simulink model "agrivoltaics_v1"  (R2025b)
settings: Solver=FixedStepAuto  StartTime=0.0  StopTime=0  FixedStep=1  RelTol=1e-3
values from neighbouring files (symbols this model uses):
  agriParams =     [agrivoltaic_multiobjective_GA_main_data.mat]    (also in agrivoltaic_multiobjective_GA_main_data_2p7_deep.mat; agrivoltaic_multiobjective_GA_main_data_berry_pop100.mat; agrivoltaic_multiobjective_GA_main_data_berry_pop50.mat; agrivoltaic_multiobjective_GA_main_data_berry_pop80.mat)
  agriVar =     [agrivoltaic_multiobjective_GA_main_data.mat]    (also in agrivoltaic_multiobjective_GA_main_data_2p7_deep.mat; agrivoltaic_multiobjective_GA_main_data_berry_pop100.mat; agrivoltaic_multiobjective_GA_main_data_berry_pop50.mat; agrivoltaic_multiobjective_GA_main_data_berry_pop80.mat)
libraries: crop_cost x1, crop_performance_module x1, environmental_module x1, pv_performance_module x1, value x1
settings Model: Creator=ciepm  LastModifiedBy=aodha

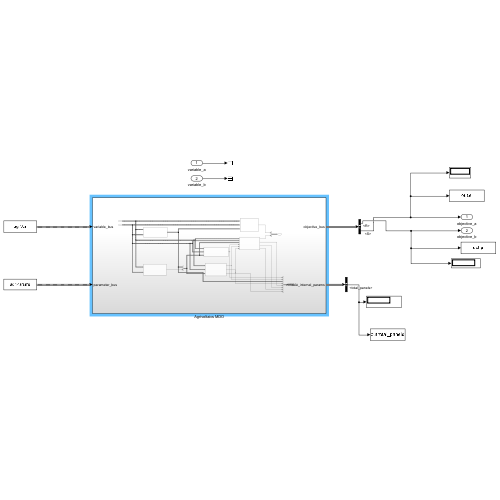
[thumbnail: Simulink's stored preview of the top-level diagram]
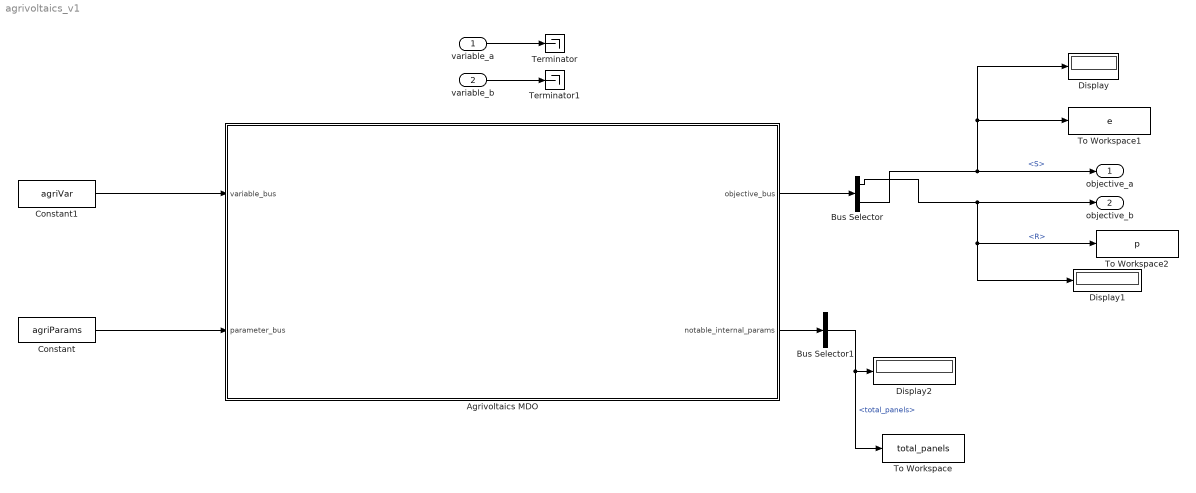
== system agrivoltaics_v1 ==
  variable_a : Inport
  variable_b : Inport  Port=2
  Agrivoltaics MDO : Subsystem
  Bus Selector : BusSelector  OutputSignals=R,S
  Bus Selector1 : BusSelector  OutputSignals=energy_per_year.total_panels
  Constant : Constant  Value=agriParams  OutDataTypeStr=Bus: params_bus
  Constant1 : Constant  Value=agriVar  OutDataTypeStr=Bus: var_bus
  Display : Display
  Display1 : Display
  Display2 : Display
  Terminator : Terminator
  Terminator1 : Terminator
  To Workspace : ToWorkspace  VariableName=total_panels  SaveFormat=Timeseries  SampleTime=-1
  To Workspace1 : ToWorkspace  VariableName=e  SaveFormat=Timeseries  SampleTime=-1
  To Workspace2 : ToWorkspace  VariableName=p  SaveFormat=Timeseries  SampleTime=-1
  objective_a : Outport
  objective_b : Outport  Port=2
  wires:
  Agrivoltaics MDO/1(objective_bus) -> Bus Selector/1
  Bus Selector/2 -> objective_a/1, To Workspace1/1, Display/1  "<S>"
  Bus Selector/1 -> objective_b/1, To Workspace2/1, Display1/1  "<R>"
  variable_a/1 -> Terminator/1
  variable_b/1 -> Terminator1/1
  Constant1/1 -> Agrivoltaics MDO/1(variable_bus)
  Agrivoltaics MDO/2(notable_internal_params) -> Bus Selector1/1
  Bus Selector1/1 -> Display2/1, To Workspace/1  "<total_panels>"
  Constant/1 -> Agrivoltaics MDO/2(parameter_bus)

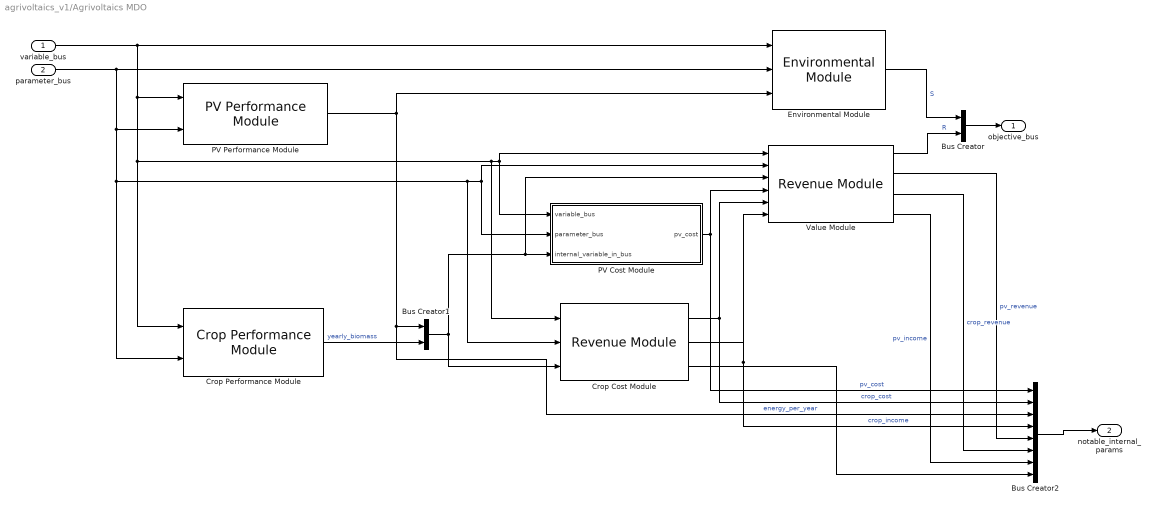
== system agrivoltaics_v1/Agrivoltaics MDO ==
  variable_bus : Inport
  parameter_bus : Inport  Port=2
  Bus Creator : BusCreator  Inputs=2
  Bus Creator1 : BusCreator  Inputs=2
  Bus Creator2 : BusCreator  Inputs=8
  Crop Cost Module : crop_cost/Revenue Module  SystemSampleTime=-1  VariantActivationTime=update diagram  EmptyChoice=off  PassThrough=off  PassThroughVariantControl=(default)  EmptyChoiceVariantControl=(default)  AllowFlexibleInterface=on  Latency=0  AutoFrameSizeCalculation=off
  Crop Performance Module : crop_performance_module/Crop Performance Module  SystemSampleTime=-1  VariantActivationTime=update diagram  EmptyChoice=off  PassThrough=off  PassThroughVariantControl=(default)  EmptyChoiceVariantControl=(default)  AllowFlexibleInterface=on  Latency=0  AutoFrameSizeCalculation=off
  Environmental Module : environmental_module/Environmental Module  SystemSampleTime=-1  VariantActivationTime=update diagram  EmptyChoice=off  PassThrough=off  PassThroughVariantControl=(default)  EmptyChoiceVariantControl=(default)  AllowFlexibleInterface=on  Latency=0  AutoFrameSizeCalculation=off
  PV Cost Module : Subsystem  AncestorBlock=pv_cost/Revenue Module
  PV Performance Module : pv_performance_module/PV Performance Module  SystemSampleTime=-1  VariantActivationTime=update diagram  EmptyChoice=off  PassThrough=off  PassThroughVariantControl=(default)  EmptyChoiceVariantControl=(default)  AllowFlexibleInterface=on  Latency=0  AutoFrameSizeCalculation=off
  Value Module : value/Revenue Module  SystemSampleTime=-1  VariantActivationTime=update diagram  EmptyChoice=off  PassThrough=off  PassThroughVariantControl=(default)  EmptyChoiceVariantControl=(default)  AllowFlexibleInterface=on  Latency=0  AutoFrameSizeCalculation=off
  objective_bus : Outport
  notable_internal_params : Outport  Port=2
  wires:
  variable_bus/1 -> Crop Performance Module/1, Crop Cost Module/1, PV Cost Module/1(variable_bus), Value Module/1, PV Performance Module/1, Environmental Module/1
  parameter_bus/1 -> Crop Performance Module/2, Crop Cost Module/2, Value Module/2, PV Cost Module/2(parameter_bus), PV Performance Module/2, Environmental Module/2
  Crop Performance Module/1 -> Bus Creator1/2  "yearly_biomass"
  Bus Creator/1 -> objective_bus/1
  Environmental Module/1 -> Bus Creator/1  "S"
  Value Module/1 -> Bus Creator/2  "R"
  PV Performance Module/1 -> Bus Creator2/3, Bus Creator1/1, Environmental Module/3  "energy_per_year"
  Bus Creator1/1 -> Value Module/3, PV Cost Module/3(internal_variable_in_bus), Crop Cost Module/3
  Bus Creator2/1 -> notable_internal_params/1
  PV Cost Module/1(pv_cost) -> Bus Creator2/1, Value Module/4  "pv_cost"
  Crop Cost Module/1 -> Bus Creator2/2, Value Module/5  "crop_cost"
  Crop Cost Module/2 -> Bus Creator2/4, Value Module/6  "crop_income"
  Value Module/2 -> Bus Creator2/5  "pv_revenue"
  Value Module/3 -> Bus Creator2/6  "crop_revenue"
  Value Module/4 -> Bus Creator2/7  "pv_income"
  Crop Cost Module/3 -> Bus Creator2/8

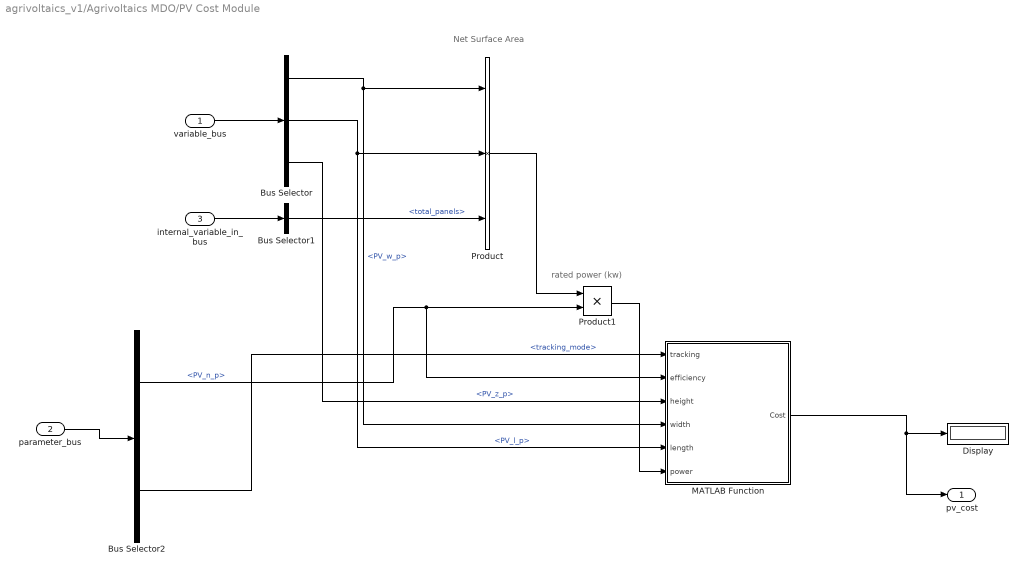
== system agrivoltaics_v1/Agrivoltaics MDO/PV Cost Module ==
  note: rated power (kw)
  note: Net Surface Area
  variable_bus : Inport
  parameter_bus : Inport  Port=2
  internal_variable_in_bus : Inport  Port=3
  Bus Selector : BusSelector  OutputSignals=PV_w_p,PV_l_p,PV_z_p
  Bus Selector1 : BusSelector  OutputSignals=energy_per_year.total_panels
  Bus Selector2 : BusSelector  OutputSignals=PV_n_p,tracking_mode
  Display : Display
  MATLAB Function : MATLAB Function  TreatAsAtomicUnit=on
  Product : Product  Inputs=3
  Product1 : Product
  pv_cost : Outport
  wires:
  variable_bus/1 -> Bus Selector/1
  parameter_bus/1 -> Bus Selector2/1
  internal_variable_in_bus/1 -> Bus Selector1/1
  Bus Selector2/1 -> MATLAB Function/2(efficiency), Product1/2  "<PV_n_p>"
  Bus Selector1/1 -> Product/3  "<total_panels>"
  Bus Selector2/2 -> MATLAB Function/1(tracking)  "<tracking_mode>"
  Bus Selector/1 -> MATLAB Function/4(width), Product/1  "<PV_w_p>"
  Bus Selector/2 -> MATLAB Function/5(length), Product/2  "<PV_l_p>"
  MATLAB Function/1(Cost) -> pv_cost/1, Display/1
  Product/1 -> Product1/1
  Product1/1 -> MATLAB Function/6(power)
  Bus Selector/3 -> MATLAB Function/3(height)  "<PV_z_p>"

== matlab function agrivoltaics_v1/Agrivoltaics MDO/PV Cost Module/MATLAB Function ==
  data: tracking input; Cost output; efficiency input; height input; width input; length input; power input
function Cost = fcn(tracking, efficiency, height, width, length, power)
    % Initialize output
    Cost = 0;

    % Tell Simulink to treat the external file as a Black Box
    coder.extrinsic('runEconomicModel');

    % Call the file. Simulink won't look inside, so no errors!
    Cost = runEconomicModel(tracking, efficiency, height, width, length, power);
end
